simulink model "Chast2"  (Simulink 4.00)
settings: Solver=ode45  StartTime=0.0  StopTime=10.0  RelTol=1e-3
settings Model: LastModifiedBy=user

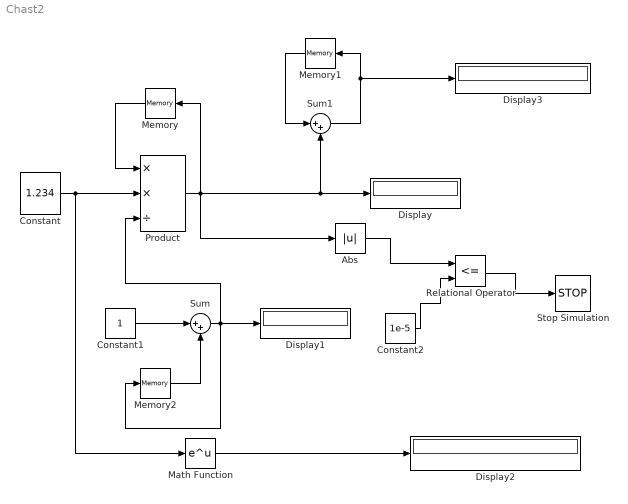
== system Chast2 ==
  Abs : Abs  SaturateOnIntegerOverflow=on
  Constant : Constant  Value=1.234
  Constant1 : Constant  Value=1
  Constant2 : Constant  Value=1e-5
  Display{,1..3} (4 alike) : Display
      Display settings: Format=short
      Display1 settings: Format=short
  Math Function : Math  Operator=exp  OutputSignalType=auto
  Memory : Memory  Orientation=left  X0=1  InheritSampleTime=off
      settings: RTWStateStorageClass=Auto
  Memory1 : Memory  Orientation=left  X0=1  InheritSampleTime=off
      settings: RTWStateStorageClass=Auto
  Memory2 : Memory  X0=0  InheritSampleTime=off
      settings: RTWStateStorageClass=Auto
  Product : Product  Inputs=**/  Multiplication=Element-wise(.*)  SaturateOnIntegerOverflow=on
  Relational Operator : RelationalOperator  Operator=<=
  Stop Simulation : Stop
  Sum : Sum  Inputs=|++  SaturateOnIntegerOverflow=on
  Sum1 : Sum  Inputs=|++  SaturateOnIntegerOverflow=on
  wires:
  Constant/1 -> Math Function/1, Product/2
  Math Function/1 -> Display2/1
  Constant1/1 -> Sum/1
  Memory2/1 -> Sum/2
  Memory/1 -> Product/1
  Product/1 -> Memory/1, Display/1, Sum1/2, Abs/1
  Memory1/1 -> Sum1/1
  Sum1/1 -> Memory1/1, Display3/1
  Sum/1 -> Memory2/1, Display1/1, Product/3
  Abs/1 -> Relational Operator/1
  Constant2/1 -> Relational Operator/2
  Relational Operator/1 -> Stop Simulation/1
